simulink model "car_sim"  (R2016b)
settings: Solver=FixedStepAuto  StartTime=0.0  StopTime=duration  FixedStep=ts_car  RelTol=1e-3
values from neighbouring files (symbols this model uses):
  ts = 0.025    [forerunner_init.m]
libraries: simulink x1
settings Model: Creator=Misi  LastModifiedBy=nagym

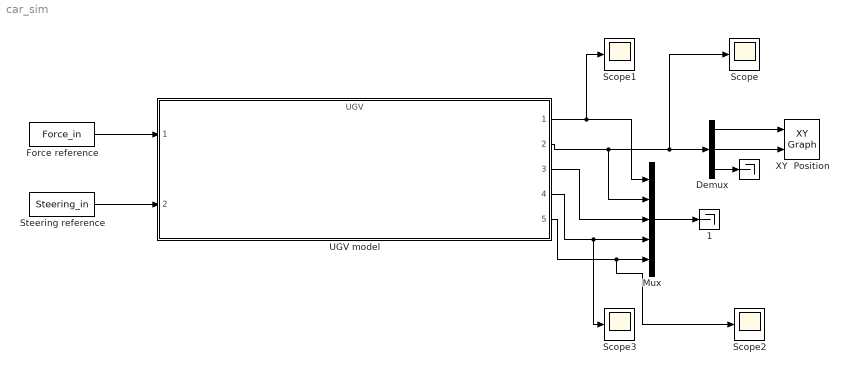
== system car_sim ==
  " " : Terminator
  " 1" : Terminator
  Demux : Demux  Outputs=3
  "Force reference " : FromWorkspace  VariableName=Force_in  SampleTime=ts
  Mux : Mux  Inputs=5
  Scope{,1..3} (4 alike) : Scope
  Steering reference : FromWorkspace  VariableName=Steering_in  SampleTime=ts
  UGV model : ModelReference  ModelNameDialog=UGV  SimulationMode=Normal  ModelReferenceVersion=1.49
  XY 	Position : simulink/Sinks/XY Graph  xmin=-30  xmax=30  ymin=-30  ymax=30  st=-1
  wires:
  "Force reference "/1 -> UGV model/1
  Steering reference/1 -> UGV model/2
  UGV model/2 -> Mux/2, Scope/1, Demux/1
  Demux/1 -> XY 	Position/1
  Demux/2 -> XY 	Position/2
  UGV model/1 -> Scope1/1, Mux/1
  UGV model/3 -> Mux/3
  UGV model/4 -> Scope3/1, Mux/4
  Demux/3 -> " "/1
  UGV model/5 -> Scope2/1, Mux/5
  Mux/1 -> " 1"/1
